simulink model "LunarLanderPolePlacementAndObserver"  (R2022b)
settings: Solver=VariableStepAuto  StartTime=0.0  StopTime=40  RelTol=1e-3
undefined symbols (not defined in the file): A, B, C, Kp, L
settings Model: Creator=marco  LastModifiedBy=marco

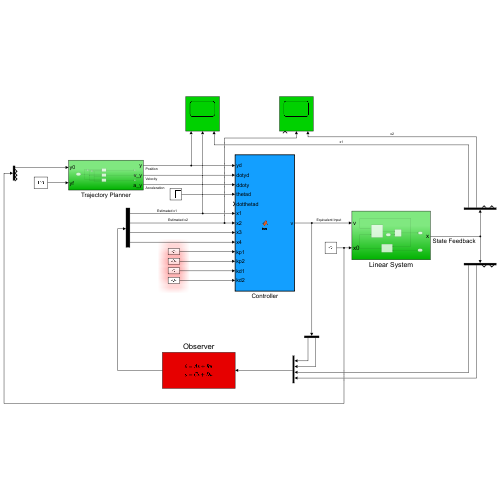
[thumbnail: Simulink's stored preview of the top-level diagram]
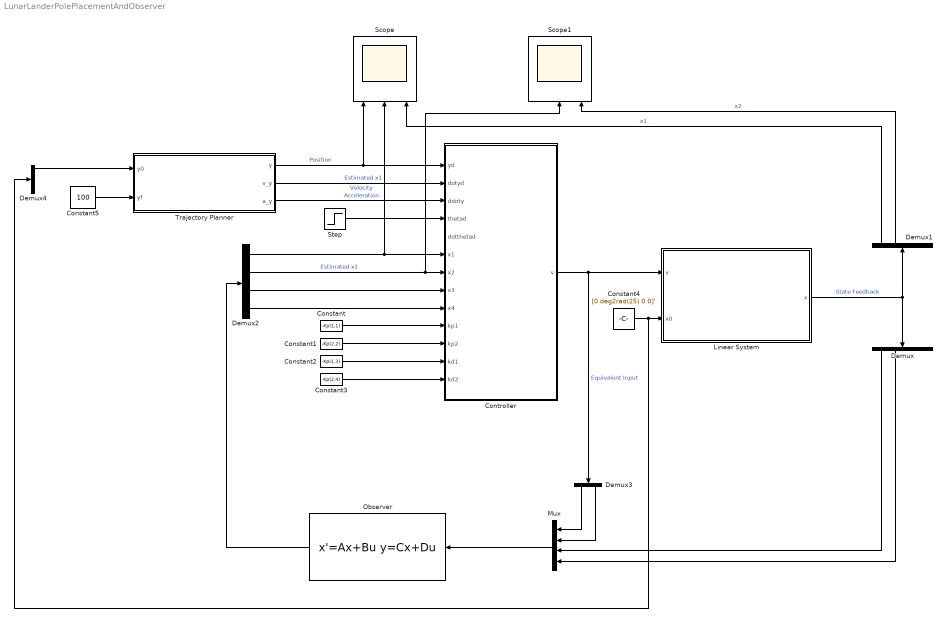
== system LunarLanderPolePlacementAndObserver ==
  Constant : Constant  Value=-Kp(1,1)
  Constant1 : Constant  Value=-Kp(2,2)
  Constant2 : Constant  Value=-Kp(1,3)
  Constant3 : Constant  Value=-Kp(2,4)
  Constant4 : Constant  Value=[0 deg2rad(25) 0 0]'
  Constant5 : Constant  Value=100
  Controller : MATLAB Function  TreatAsAtomicUnit=on
  Demux{,1..2,4} (4 alike) : Demux
  Demux3 : Demux  Outputs=2
  Linear System : Subsystem
  Mux : Mux
  Observer : StateSpace  A=A-L*C  B=[B L]  C=eye(4)  D=zeros(4)  InitialCondition=0
  Scope : Scope  NumInputPorts=3
  Scope1 : Scope  NumInputPorts=3
  Step : Step  After=deg2rad(0)  SampleTime=0
  Trajectory Planner : Subsystem
  wires:
  Linear System/1(x) -> Demux1/1, Demux/1  "State Feedback"
  Constant/1 -> Controller/10(kp1)
  Constant1/1 -> Controller/11(kp2)
  Constant2/1 -> Controller/12(kd1)
  Constant3/1 -> Controller/13(kd2)
  Trajectory Planner/1(y) -> Controller/1(yd), Scope/1  "Position"
  Controller/1(v) -> Demux3/1, Linear System/1(v)  "Equivalent Input"
  Mux/1 -> Observer/1
  Observer/1 -> Demux2/1
  Demux/1 -> Mux/3
  Demux/2 -> Mux/4
  Demux3/1 -> Mux/1
  Demux3/2 -> Mux/2
  Demux2/1 -> Controller/6(x1), Scope/2  "Estimated x1"
  Demux2/2 -> Controller/7(x2), Scope1/2  "Estimated x2"
  Demux2/4 -> Controller/9(x4)
  Demux2/3 -> Controller/8(x3)
  Step/1 -> Controller/4(thetad)
  Trajectory Planner/2(v_y) -> Controller/2(dotyd)  "Velocity"
  Trajectory Planner/3(a_y) -> Controller/3(ddoty)  "Acceleration"
  Demux1/1 -> Scope/3  "x1"
  Demux1/2 -> Scope1/3  "x2"
  Demux4/1 -> Trajectory Planner/1(y0)
  Constant4/1 -> Demux4/1, Linear System/2(x0)
  Constant5/1 -> Trajectory Planner/2(yf)

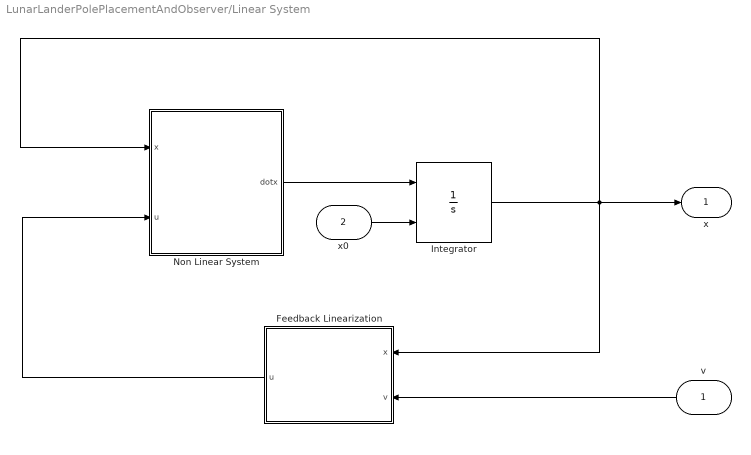
== system LunarLanderPolePlacementAndObserver/Linear System ==
  v : Inport
  x0 : Inport  Port=2
  Feedback Linearization : MATLAB Function  TreatAsAtomicUnit=on
  Integrator : Integrator  InitialConditionSource=external  InitialCondition=[0 0 0 0]'
  Non Linear System : MATLAB Function  TreatAsAtomicUnit=on
  x : Outport
  wires:
  Feedback Linearization/1(u) -> Non Linear System/2(u)
  Integrator/1 -> Non Linear System/1(x), x/1, Feedback Linearization/1(x)
  v/1 -> Feedback Linearization/2(v)
  Non Linear System/1(dotx) -> Integrator/1
  x0/1 -> Integrator/2

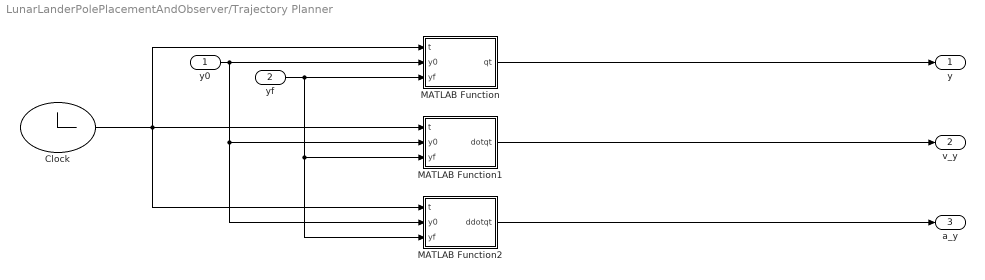
== system LunarLanderPolePlacementAndObserver/Trajectory Planner ==
  y0 : Inport
  yf : Inport  Port=2
  Clock : Clock
  MATLAB Function : MATLAB Function  TreatAsAtomicUnit=on
  MATLAB Function1 : MATLAB Function  TreatAsAtomicUnit=on
  MATLAB Function2 : MATLAB Function  TreatAsAtomicUnit=on
  y : Outport
  v_y : Outport  Port=2
  a_y : Outport  Port=3
  wires:
  MATLAB Function/1(qt) -> y/1
  MATLAB Function1/1(dotqt) -> v_y/1
  MATLAB Function2/1(ddotqt) -> a_y/1
  Clock/1 -> MATLAB Function1/1(t), MATLAB Function2/1(t), MATLAB Function/1(t)
  y0/1 -> MATLAB Function1/2(y0), MATLAB Function2/2(y0), MATLAB Function/2(y0)
  yf/1 -> MATLAB Function1/3(yf), MATLAB Function2/3(yf), MATLAB Function/3(yf)

== matlab function LunarLanderPolePlacementAndObserver/Linear System/Feedback Linearization ==
  data: x input; v input; u output
function u = fcn(x, v)

g = 1.62;
m = 23000;
J = 100000;
c = 1000;

Q = [sin(x(2))/m cos(x(2))/m;4/J 0]
Qinv = Q^-1

A = [-(g-c*x(3)/m); 0]
ueq = Qinv*(-A+v)

u = [ueq(1); ueq(2)];

== matlab function LunarLanderPolePlacementAndObserver/Linear System/Non Linear System ==
  data: x input; u input; dotx output
function dotx  = fcn(x, u)

g = 1.62;
m = 23000;
J = 100000;
c = 1000;

y = x(1)
theta = x(2)
v = x(3)
w = x(4)

doty = v
dottheta = w
dotv = (u(1)*sin(theta)+u(2)*cos(theta)-m*g-c*v)/m
dotw = 4*u(1)/J

dotx = [doty, dottheta, dotv, dotw]';

== matlab function LunarLanderPolePlacementAndObserver/Controller ==
  data: yd input; dotyd input; ddoty input; thetad input; dotthetad input; x1 input; x2 input; x3 input; x4 input; v output; kp1 input; kp2 input; kd1 input; kd2 input
function v = fcn(yd, dotyd, ddoty, thetad, dotthetad, x1, x2, x3, x4, kp1, kp2, kd1, kd2)

v1 = kp1*(x1-yd) + kd1*(x3-dotyd) + ddoty
v2 = kp2*(x2-thetad) + kd2*(x4-dotthetad) + 0

v = [v1; v2]

== matlab function LunarLanderPolePlacementAndObserver/Trajectory Planner/MATLAB Function ==
  data: t input; qt output; y0 input; yf input
function qt = fcn(t, y0, yf)

tf = 20 %s
dotqc = 8 %m/s
qi = y0 %m - valore integratore per y_0
qf = yf %m

tc = tf - (qf - qi)/dotqc

ddotqc = dotqc/tc

q1 = qi + 0.5 * ddotqc * t^2;
q2 = qi + ddotqc*tc*(t-tc/2);
q3 = qi + ddotqc*tc*(tf-tc-tc/2) + dotqc*(t-(tf-tc))-0.5*ddotqc*(t-(tf-tc))^2;

if t>=0 && t<=tc
    qt = q1
elseif t>tc && t<=(tf-tc)
    qt = q2
elseif t>(tf-tc) && t<=tf
    qt = q3
elseif t>tf
    qt = yf
else 
    qt = 0
end

== matlab function LunarLanderPolePlacementAndObserver/Trajectory Planner/MATLAB Function1 ==
  data: t input; dotqt output; y0 input; yf input
function dotqt = fcn(t, y0, yf)

tf = 20 %s
dotqc = 8 %m/s
qi = y0 %m - valore integratore per y_0
qf = yf %m

tc = tf - (qf - qi)/dotqc

ddotqc = dotqc/tc

dotq1 = ddotqc*t;
dotq2 = dotqc;
dotq3 = dotqc-ddotqc*(t-(tf-tc));

if t>=0 && t<=tc
    dotqt = dotq1
elseif t>tc && t<=(tf-tc)
    dotqt = dotq2
elseif t>(tf-tc) && t<=tf
    dotqt = dotq3
else 
    dotqt = 0
end

== matlab function LunarLanderPolePlacementAndObserver/Trajectory Planner/MATLAB Function2 ==
  data: t input; ddotqt output; y0 input; yf input
function ddotqt = fcn(t, y0, yf)

tf = 20 %s
dotqc = 8 %m/s
qi = y0 %m - valore integratore per y_0
qf = yf %m

tc = tf - (qf - qi)/dotqc

ddotqc = dotqc/tc

ddotq1 = ddotqc;
ddotq2 = 0;
ddotq3 = -ddotqc;

if t>=0 && t<=tc
    ddotqt = ddotq1
elseif t>tc && t<=(tf-tc)
    ddotqt = ddotq2
elseif t>(tf-tc) && t<=tf
    ddotqt = ddotq3
else 
    ddotqt = 0
end
